simulink model "dab_converter"  (R2022b)
settings: Solver=VariableStepAuto  StartTime=0.0  StopTime=1  RelTol=1e-3
libraries: spsMosfetLib x8, spsVoltageMeasurementLib x3, spsCurrentMeasurementLib x2, spsSeriesRLCBranchLib x2, spsDCVoltageSourceLib x1, spsLinearTransformerLib x1, sps_lib x1
settings Model: Creator=vemur  LastModifiedBy=vemur

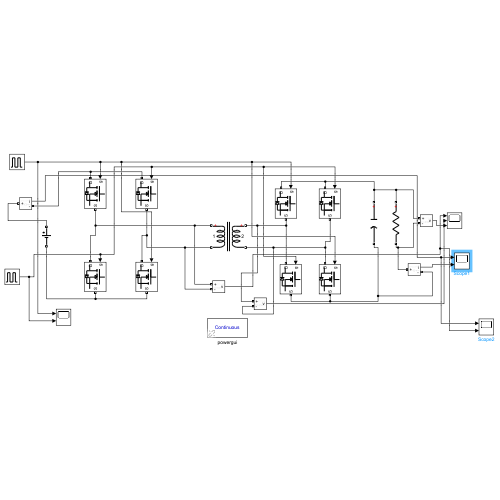
[thumbnail: Simulink's stored preview of the top-level diagram]
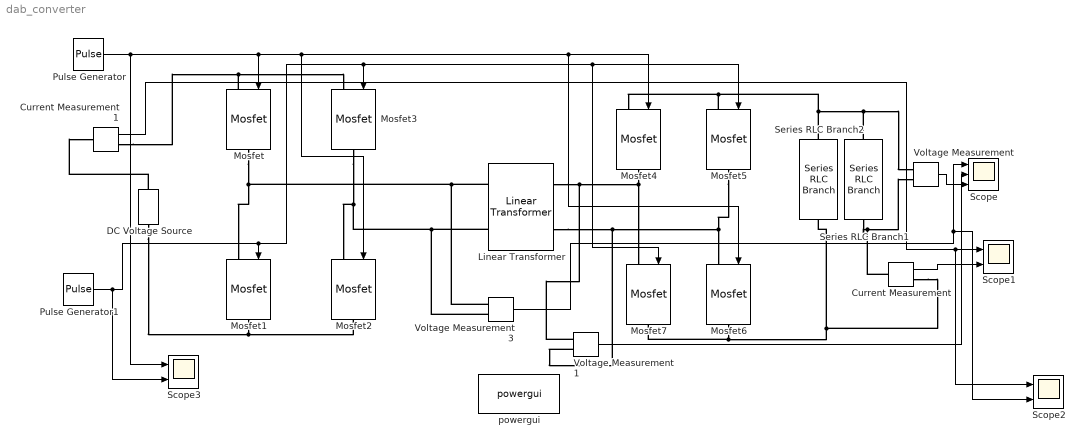
== system dab_converter ==
  Current Measurement : spsCurrentMeasurementLib/Current Measurement  PhasorSimulation=off  OutputType=Complex  PSBequivalent=0
  Current Measurement1 : spsCurrentMeasurementLib/Current Measurement  PhasorSimulation=off  OutputType=Complex  PSBequivalent=0
  DC Voltage Source : spsDCVoltageSourceLib/DC Voltage Source  Amplitude=400  Measurements=None
  Linear Transformer : spsLinearTransformerLib/Linear Transformer  UNITS=SI  NominalPower=[ 10000 100000]  winding1=[400 0 0]  winding2=[400 0 0]  ThreeWindings=off  winding3=[3.15e+05 0.7938 0.084225]  RmLm=[1.0805e+05 2866]  Measurements=None  DataType=on
  Mosfet{,1..7} (8 alike) : spsMosfetLib/Mosfet  Ron=0.1  Lon=0  Rd=0.01  Vfd=0  IC=0  Rs=1e5  Cs=inf  Measurements=off
  Pulse Generator : DiscretePulseGenerator  PulseType=Time based  Amplitude=10  Period=1e-5  PulseWidth=48
  Pulse Generator1 : DiscretePulseGenerator  PulseType=Time based  Amplitude=10  Period=1e-5  PulseWidth=48  PhaseDelay=5e-6
  Scope : Scope  NumInputPorts=3
  Scope1 : Scope  NumInputPorts=2
  Scope2 : Scope  NumInputPorts=2
  Scope3 : Scope  NumInputPorts=2
  Series RLC Branch1 : spsSeriesRLCBranchLib/Series RLC Branch  LConnTagsString=__new0  RConnTagsString=__new0  BranchType=R  Resistance=50  Inductance=1e-3  SetiL0=off  InitialCurrent=0  Capacitance=1e-6  Setx0=off  InitialVoltage=0  Measurements=None
  Series RLC Branch2 : spsSeriesRLCBranchLib/Series RLC Branch  LConnTagsString=__new0  RConnTagsString=__new0  BranchType=C  Resistance=50  Inductance=1e-3  SetiL0=off  InitialCurrent=0  Capacitance=1000e-6  Setx0=off  InitialVoltage=0  Measurements=None
  Voltage Measurement : spsVoltageMeasurementLib/Voltage Measurement  PhasorSimulation=off  OutputType=Complex  PSBequivalent=0
  Voltage Measurement1 : spsVoltageMeasurementLib/Voltage Measurement  PhasorSimulation=off  OutputType=Complex  PSBequivalent=0
  Voltage Measurement3 : spsVoltageMeasurementLib/Voltage Measurement  PhasorSimulation=off  OutputType=Complex  PSBequivalent=0
  powergui : sps_lib/powergui  Priority=1  SimulationMode=Continuous  SampleTime=50e-6  frequency=60  Iterations=50  frequencyindice=0  Pbase=100e6  ErrMax=1e-4  UnitsV=kV  UnitsW=MW  buscounter=0  FunctionMessages=off  echomessages=off  EnableUseOfTLC=off  CurrentSourceSwitches=off  DisableSnubberDevices=off  DisableRonSwitches=off  DisableVfSwitches=off  DisplayEquations=off  AutomaticDiscreteSolvers=off  SolverType=Tustin/Backward Euler (TBE)  Interpol=off  ExternalGateDelay=off  methode=off  Ts=100  x0status=blocks  SPID=on  SwTol=0  HookPort=off  NonlinearTolerance=1e-4  nMaxIteration=100  ContinueOnMaxIteration=off  RestoreLinks=warning  ResistiveCurrentMeasurement=off  Frange=[0:2:500]  Ylog=off  Xlog=on  ShowGrid=off  save=off  variable=ZData  structure=0  ZoomFFT=off  StartTime=0.0  cycles=1  DisplayStyle=1  fundamental=60  FreqAxis=off  MaxFrequency=1000  frequencyindicesteady=1  RmsSteady=1  display=off
  wires:
  Voltage Measurement/1 -> Scope/3
  Pulse Generator/1 -> Mosfet6/1, Mosfet4/1, Mosfet2/1, Mosfet/1, Scope3/1
  Pulse Generator1/1 -> Scope3/2, Mosfet7/1, Mosfet5/1, Mosfet3/1, Mosfet1/1
  Voltage Measurement3/1 -> Scope2/2, Scope/1
  Voltage Measurement1/1 -> Scope/2
  Current Measurement1/1 -> Scope2/1, Scope1/1
  Current Measurement/1 -> Scope1/2
  connections:
  Series RLC Branch1/RConn1 -- Current Measurement/LConn1 -- Voltage Measurement/LConn2
  Mosfet/LConn1 -- Current Measurement1/RConn1 -- Mosfet3/LConn1
  Mosfet/RConn1 -- Voltage Measurement3/LConn1 -- Linear Transformer/LConn1 -- Mosfet1/LConn1
  Mosfet3/RConn1 -- Voltage Measurement3/LConn2 -- Linear Transformer/LConn2 -- Mosfet2/LConn1
  Mosfet1/RConn1 -- Mosfet2/RConn1 -- DC Voltage Source/LConn1
  Series RLC Branch1/LConn1 -- Mosfet4/LConn1 -- Mosfet5/LConn1 -- Series RLC Branch2/LConn1 -- Voltage Measurement/LConn1
  Mosfet4/RConn1 -- Voltage Measurement1/LConn1 -- Linear Transformer/RConn1 -- Mosfet7/LConn1
  Mosfet5/RConn1 -- Voltage Measurement1/LConn2 -- Linear Transformer/RConn2 -- Mosfet6/LConn1
  Mosfet6/RConn1 -- Mosfet7/RConn1 -- Current Measurement/RConn1 -- Series RLC Branch2/RConn1
  DC Voltage Source/RConn1 -- Current Measurement1/LConn1
